simulink model "Demo_V2XStats_Intersection_1_cs"  (R2014b)
settings: Solver=FixedStepDiscrete  SolverMode=SingleTasking  StartTime=0.0  StopTime=10  FixedStep=1/20  RelTol=1e-3
PreLoadFcn:
  | mbxruntime.callbacks.PreLoadFcn(bdroot);
  | check_NUTS_defined
  | model_closed = 0;
  | assignin('base',['model_closed_' bdroot],false);
PostLoadFcn:
  | mbxruntime.callbacks.PostLoadFcn(bdroot);
InitFcn:
  | mbxruntime.callbacks.InitFcn(bdroot);
StartFcn:
  | mbxruntime.callbacks.StartFcn(bdroot);
StopFcn:
  | mbxruntime.callbacks.StopFcn(bdroot);;
  | 
  | PostProcessing
  | 
model workspace: external: MAT-File .\Demo_V2XStats_Intersection_1_cs_hws.mat (data not in the file)
undefined symbols (not defined in the file or in its folder): InitializeBus, mbxruntime, tabledata
undefined symbols (not defined in the file): Demo_V2XStats_Intersection_1_cs_022fa72960d02a99, Demo_V2XStats_Intersection_1_cs_0667b7440011464a, Demo_V2XStats_Intersection_1_cs_0a717f3b1f82dce8, Demo_V2XStats_Intersection_1_cs_1912d0ac773e0614, Demo_V2XStats_Intersection_1_cs_1b4820430dd12493, Demo_V2XStats_Intersection_1_cs_3bba87328ee67e0a, Demo_V2XStats_Intersection_1_cs_467d7b57b3557fc2, Demo_V2XStats_Intersection_1_cs_534bad308c560994, Demo_V2XStats_Intersection_1_cs_58d6839509a0e403, Demo_V2XStats_Intersection_1_cs_7e2090151d7b4087, Demo_V2XStats_Intersection_1_cs_9888c4f7e8bf41a4, Demo_V2XStats_Intersection_1_cs_a103b1f27004d7b9, Demo_V2XStats_Intersection_1_cs_dde6e9b2bb85eae6, Demo_V2XStats_Intersection_1_cs_fcdd4688b7d5d124
libraries: simulink x5, PreScanSimulinkLibrary x4, PreScanUsefulBlocks x1, simulink_extras x1
(part 1 of 3)
CloseFcn:
  | mbxruntime.callbacks.CloseFcn(bdroot);
  | evalin('base',['clear model_closed_' bdroot]);
  | model_closed = 1;
settings Model: Creator=PRESCAN  LastModifiedBy=stq0ee
settings DataIOCC: SignalLoggingSaveFormat=ModelDataLogs
settings OptimizationCC: InlineParams=on  ExpressionDepthLimit=2147483647  InitFltsAndDblsToZero=on
settings DebuggingCC: SaveWithParameterizedLinksMsg=none  UnderspecifiedInitializationDetection=Classic  MergeDetectMultiDrivingBlocksExec=none  SignalResolutionControl=TryResolveAllWithWarning  SolverPrmCheckMsg=none  MultiTaskDSMMsg=warning  MultiTaskCondExecSysMsg=none  FcnCallInpInsideContextMsg=UseLocalSettings  StateNameClashWarn=warning
settings ModelReferenceCC: UpdateModelReferenceTargets=IfOutOfDate
settings SFSimCC: SimParseCustomCode=off
settings SFSimCC: SimCustomHeaderCode=|
  | #include "prescan.h"
  | #include "prescan_platform.h"
  | #include "prescan_v2x_data.h"
settings RTWCC: IncludeERTFirstTime=on
settings GRTTargetCC: TargetFcnLib=ansi_tfl_tmw.mat  CombineOutputUpdateFcns=off  GRTInterface=on

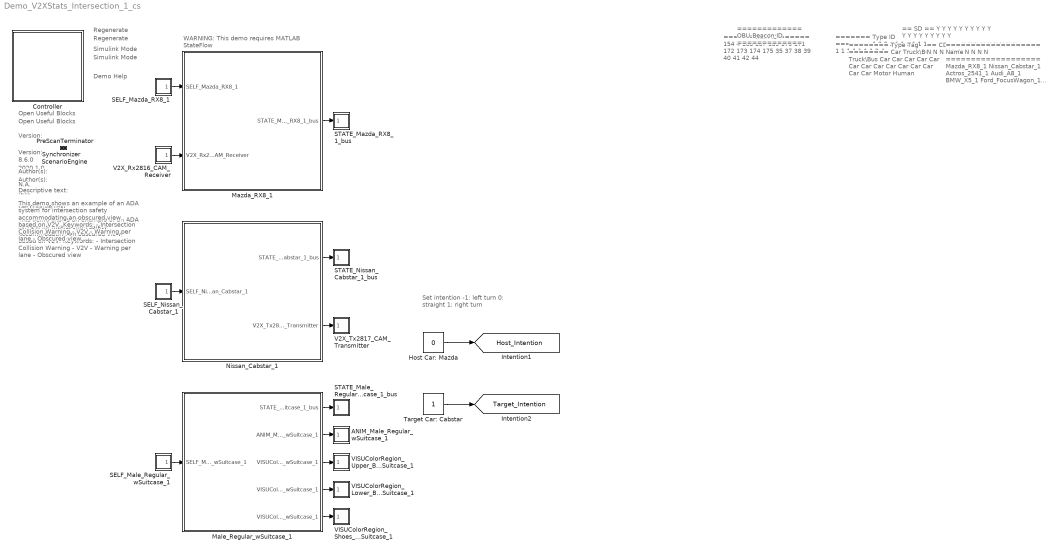
== system Demo_V2XStats_Intersection_1_cs ==
  note: Regenerate
  note: Simulink Mode
  note: Open Useful Blocks
  note: 2020.1.0
  note: Version:
  note: Author(s):
  note: N.A.
  note: Descriptive text:
  note: This demo shows an example of an
      | ADA system for intersection
      | safety accommodating an obscured
      | view, based on V2V.
      |
      |
      |
      | Keywords:
      |
      | - Intersection Collision Warning
      |
      | - V2V
      |
      | - Warning per lane
      |
      | - Obscured view
  note: 8.6.0
  note: Demo Help
  note: WARNING:
      | This demo requires MATLAB StateFlow
  note: Set intention
      | -1: left turn
      | 0: straight
      | 1: right turn
  note: This demo shows an example of an
      | ADA system for intersection
      | safety accommodating an obscured
      | view, based on V2V.
      |
      |
      |
      | Keywords:
      |
      | - Intersection Collision Warning
      |
      | - V2V
      |
      | - Warning per lane
      |
      | - Obscured view
  note: Descriptive text:
  note: N.A.
  note: Author(s):
  note: Version:
  note: Open Useful Blocks
  note: Simulink Mode
  note: Regenerate
  note: ======
      | Num ID
      | ======
      | 154
      | 4
      | 168
      | 167
      | 169
      | 170
      | 171
      | 172
      | 173
      | 174
      | 175
      | 35
      | 37
      | 38
      | 39
      | 40
      | 41
      | 42
      | 44
  note: =============
      | OBU-Beacon ID
      | =============
  note: =======
      | Type ID
      | =======
      | 1
      | 3
      | 3
      | 1
      | 1
      | 1
      | 1
      | 1
      | 1
      | 1
      | 1
      | 1
      | 1
      | 1
      | 1
      | 1
      | 1
      | 2
      | 4
  note: ========
      | Type Tag
      | ========
      | Car
      | Truck\Bus
      | Truck\Bus
      | Car
      | Car
      | Car
      | Car
      | Car
      | Car
      | Car
      | Car
      | Car
      | Car
      | Car
      | Car
      | Car
      | Car
      | Motor
      | Human
  note: ==
      | SD
      | ==
      | Y
      | Y
      | Y
      | Y
      | Y
      | Y
      | Y
      | Y
      | Y
      | Y
      | Y
      | Y
      | Y
      | Y
      | Y
      | Y
      | Y
      | Y
      | Y
  note: ==
      | CD
      | ==
      | N
      | N
      | N
      | N
      | N
      | N
      | N
      | N
      | N
      | N
      | N
      | N
      | N
      | N
      | N
      | N
      | N
      | N
      | N
  note: ===================
      | Name
      | ===================
      | Mazda_RX8_1
      | Nissan_Cabstar_1
      | Actros_2541_1
      | Audi_A8_1
      | BMW_X5_1
      | Ford_FocusWagon_1
      | Fiat_Bravo_1
      | Toyota_Previa_2
      | Citroen_C3_1
      | BMW_Z3_1
      | Ford_FocusWagon_2
      | Audi_A8_2
      | BMW_X5_2
      | Ford_FocusWagon_3
      | Mazda_RX8_2
      | Mazda_RX8_3
      | Ford_Fiesta_1
      | Honda_Pan_European_1
      | Male_Regular_wSuitcase_1
  ANIM_Male_Regular_wSuitcase_1 : Subsystem  Tag=actuator/AnimationOutport  Priority=0  LoadFcn=load('PreScanAnimActuatorData.mat')  mask(PreScan Sink Block: State Animation){}
      mask help: The Human Animation port allows the human to walk, run or bend
      settings: OpenFcn=open_system([gcb '/Actuator'],'mask')
      mask Help: eval('openHelp(239)')
      mask Display: image(imread('HumanAnimated.jpg'))
  Controller : Subsystem  Description=8A3CD2955739A82C886C20AE3E253D78460D53180EE2C1B14CC08DF75A70BE77  Priority=-1  LoadFcn=load PreScanControllerData  mask(PreScan Simulation Controller){prescanversion='2020.1.0', ModelReferencing=off, TimeStep=1/20, ControlMode=0, PreScanExecutionMode=on, ControllerCount=0, ControllerIndex=0, ControllerOptions=''}
      mask prompts: prescanversion "PreScan Version"; ModelReferencing "Use Model Referencing"; TimeStep "Upload Period [s]"; ControlMode "Control Mode"; PreScanExecutionMode "Execution Mode"; ControllerCount "Controller Count"; ControllerIndex "Controller Index"; ControllerOptions "Controller Options"
      mask help:
      | Please do not remove this block from the compilation sheet,
      | as it connects the model to the PreScan environment.
      mask init:
      | model = bdroot(gcb);
      | ExperimentFile = mbxruntime.findExperimentFile(model,true); %relative path
      | 
      | [d1, d2, d3, prescandata] = prescan_Settings();
      | ModelDepo = fullfile(prescandata,'ModelDepo'); 
      | 
      | RTmode = mbxruntime.getRTMode(model);
      | 
      | SimulationMode = get_param(bdroot,'SimulationMode');
      | if strcmp(SimulationMode, 'rapid-accelerator')
      |     SimulationMode = 'external';
      | end
      | TargetName = get_param(bdroot,'SystemTargetFile');
      settings: ModelCloseFcn=assignin('base',['model_closed_' bdroot],true);
      mask Help: eval('openHelp(812)')
      mask Display: image(imread('prescanlogo.ico'))
  Host Car: Mazda : Constant  Value=0
  Male_Regular_wSuitcase_1 : Subsystem  Tag=WorldObjectSubSystem  InitFcn=UniqueId = '2658';
      mask init:
      | modelPath = GenericModelHelper.getGenericModelFilePath('ModelDepo','Humans\MaleSuitcase\Male_wSuitcase.pgmb','86bcb677b51d2887e0050f1727544e76');imagePath = GenericModelHelper.getCompilationPicture(modelPath, 'MaleSuitcase.png');
      mask Display: image(imread(imagePath));color('white');text(0, 0, ' ID=44\n')
  Mazda_RX8_1 : Subsystem  Tag=WorldObjectSubSystem  InitFcn=UniqueId = '7';
      mask init:
      | modelPath = GenericModelHelper.getGenericModelFilePath('ModelDepo','Vehicles\Mazda_RX8\Mazda_RX8.pgmb','1e55a2e40efa576b7f4fb93bae35d605');imagePath = GenericModelHelper.getCompilationPicture(modelPath, 'Mazda_RX8_HighPoly.png');
      mask Display: image(imread(imagePath));color('white');text(0, 0, ' ID=154\n')
  Nissan_Cabstar_1 : Subsystem  Tag=WorldObjectSubSystem  InitFcn=UniqueId = '10';
      mask init:
      | modelPath = GenericModelHelper.getGenericModelFilePath('ModelDepo','Vehicles\Nissan_Cabstar\Nissan_Cabstar.pgmb','dd076fdae311093c5436e82e6c23dc23');imagePath = GenericModelHelper.getCompilationPicture(modelPath, 'Nissan_Cabstar_HighPoly.png');
      mask Display: image(imread(imagePath));color('white');text(0, 0, ' ID=4\n')
  PreScanTerminator : Subsystem  Tag=PreScanTerminator  Priority=999  LoadFcn=load PrescanTerminatorData  mask(PreScan Simulation Terminator){TimeStep=1/20}
      mask prompts: TimeStep "Upload Period [s]"
      mask help:
      | Please do not remove this block from the compilation sheet as it
      | connects the model to the PreScan environment.
      mask Help: eval('openHelp(812)')
      mask Display: image(imread('prescanlogo.ico'))
  SELF_Male_Regular_wSuitcase_1 : Subsystem  Tag=sensor/SelfPort  Priority=30  LoadFcn=load('PreScanSelfSensorData.mat')  mask(PreScan Source Block: SELF){}
      mask help:
      | The SELF port shows (state) information of the actor itself. The outputs are position in the experiment's axis system and the GPS coordinates, and the object's absolute velocity and compass heading.
      |
      | For more information, please click Help.
      settings: OpenFcn=open_system([gcb '/Sensor'],'mask')
      mask Help: eval('openHelp(462)')
      mask Display: image(imread('GPS.png'))
  SELF_Mazda_RX8_1 : Subsystem  Tag=sensor/SelfPort  Priority=30  LoadFcn=load('PreScanSelfSensorData.mat')  mask(PreScan Source Block: SELF){}
      mask help:
      | The SELF port shows (state) information of the actor itself. The outputs are position in the experiment's axis system and the GPS coordinates, and the object's absolute velocity and compass heading.
      |
      | For more information, please click Help.
      settings: OpenFcn=open_system([gcb '/Sensor'],'mask')
      mask Help: eval('openHelp(462)')
      mask Display: image(imread('GPS.png'))
  SELF_Nissan_Cabstar_1 : Subsystem  Tag=sensor/SelfPort  Priority=30  LoadFcn=load('PreScanSelfSensorData.mat')  mask(PreScan Source Block: SELF){}
      mask help:
      | The SELF port shows (state) information of the actor itself. The outputs are position in the experiment's axis system and the GPS coordinates, and the object's absolute velocity and compass heading.
      |
      | For more information, please click Help.
      settings: OpenFcn=open_system([gcb '/Sensor'],'mask')
      mask Help: eval('openHelp(462)')
      mask Display: image(imread('GPS.png'))
  STATE_Male_Regular_wSuitcase_1_bus : Subsystem  Tag=actuator/StatePort  Priority=0  LoadFcn=load('PreScanStateActuatorData.mat')  mask(PreScan Sink Block: State){}
      mask help:
      | The Actor State contains a vector signal of size (9x1), containing the following signals:
      |
      | -  Position    	(x,y,z)             	[m]
      | -  Velocity    	(vx,vy,vz)         	[m/s]
      | -  Angles       	(Roll, Pitch, Yaw)	[rad]
      |
      | The Actor state is defined in the global axis system.
      | The state is superponed on the Initial position defined in the GUI.
      |
      | For more information, please click Help.
      settings: OpenFcn=open_system([gcb '/Actuator'],'mask')
      mask Help: eval('openHelp(222)')
      mask Display: image(imread('State.png'))
  STATE_Mazda_RX8_1_bus : Subsystem  Tag=actuator/StatePort  Priority=0  LoadFcn=load('PreScanStateActuatorData.mat')  mask(PreScan Sink Block: State){}
      mask help:
      | The Actor State contains a vector signal of size (9x1), containing the following signals:
      |
      | -  Position    	(x,y,z)             	[m]
      | -  Velocity    	(vx,vy,vz)         	[m/s]
      | -  Angles       	(Roll, Pitch, Yaw)	[rad]
      |
      | The Actor state is defined in the global axis system.
      | The state is superponed on the Initial position defined in the GUI.
      |
      | For more information, please click Help.
      settings: OpenFcn=open_system([gcb '/Actuator'],'mask')
      mask Help: eval('openHelp(222)')
      mask Display: image(imread('State.png'))
  STATE_Nissan_Cabstar_1_bus : Subsystem  Tag=actuator/StatePort  Priority=0  LoadFcn=load('PreScanStateActuatorData.mat')  mask(PreScan Sink Block: State){}
      mask help:
      | The Actor State contains a vector signal of size (9x1), containing the following signals:
      |
      | -  Position    	(x,y,z)             	[m]
      | -  Velocity    	(vx,vy,vz)         	[m/s]
      | -  Angles       	(Roll, Pitch, Yaw)	[rad]
      |
      | The Actor state is defined in the global axis system.
      | The state is superponed on the Initial position defined in the GUI.
      |
      | For more information, please click Help.
      settings: OpenFcn=open_system([gcb '/Actuator'],'mask')
      mask Help: eval('openHelp(222)')
      mask Display: image(imread('State.png'))
  ScenarioEngine : Subsystem  Tag=PreScanOpenScenarioBlock  Priority=10  LoadFcn=load PrescanSynchronizeData  mask(PreScan Simulation Core Block){TimeStep=1/20}
      mask prompts: TimeStep "Timestep [s]"
      mask help:
      | Please do not remove this block from the PreScan compilation sheet,
      | as it contains essential configuration parameters for a PreScan simulation.
      settings: DeleteFcn=PreScanBlockDeleteFcn;
      mask Display: image(imread('prescanlogo.ico'))
  Synchronizer : Subsystem  Tag=PreScanSynchronizer  Priority=20  LoadFcn=load PrescanSynchronizeData  mask(PreScan Simulation Core Block){TimeStep=1/20}
      mask prompts: TimeStep "Timestep [s]"
      mask help:
      | Please do not remove this block from the PreScan compilation sheet,
      | as it contains essential configuration parameters for a PreScan simulation.
      settings: DeleteFcn=PreScanBlockDeleteFcn;
      mask Display: image(imread('prescanlogo.ico'))
  Target Car: Cabstar : Constant
  V2X_Rx2816_CAM_Receiver : Subsystem  Tag=sensor/plugin/sfun_V2X_CAM_Receiver  Priority=30  mask(V2X CAM Receiver Block){}
      mask help: V2X Block receiving a CAM message
      settings: OpenFcn=open_system([gcb '/Sensor'],'mask')
      mask Help: eval('openHelp()')
      mask Display: image(imread('V2XR_grayscale.png'))
  V2X_Tx2817_CAM_Transmitter : Subsystem  Tag=actuator/plugin/sfun_V2X_CAM_Transmitter  Priority=0  mask(V2X CAM Transmitter Block){}
      mask help: V2X Block transmitting a CAM message
      settings: OpenFcn=open_system([gcb '/Actuator'],'mask')
      mask Help: eval('openHelp()')
      mask Display: image(imread('V2XT_grayscale.png'))
  VISUColorRegion_Lower_Body_Male_Regular_wSuitcase_1 : Subsystem  Tag=actuator/ColorRegion  Priority=0  LoadFcn=load('PrescanColorData')  mask(PreScan Sink Block: VisuTextureColor){}
      mask help:
      | The VisuTextureColor block provides a way to adapt the color of a vehicle.
      |
      | For more information, please click Help.
      settings: OpenFcn=open_system([gcb '/Actuator'],'mask')
      mask Help: eval('openHelp(230)')
      mask Display: image(imread('TextureColor.png'))
  VISUColorRegion_Shoes_Male_Regular_wSuitcase_1 : Subsystem  Tag=actuator/ColorRegion  Priority=0  LoadFcn=load('PrescanColorData')  mask(PreScan Sink Block: VisuTextureColor){}
      mask help:
      | The VisuTextureColor block provides a way to adapt the color of a vehicle.
      |
      | For more information, please click Help.
      settings: OpenFcn=open_system([gcb '/Actuator'],'mask')
      mask Help: eval('openHelp(230)')
      mask Display: image(imread('TextureColor.png'))
  VISUColorRegion_Upper_Body_Male_Regular_wSuitcase_1 : Subsystem  Tag=actuator/ColorRegion  Priority=0  LoadFcn=load('PrescanColorData')  mask(PreScan Sink Block: VisuTextureColor){}
      mask help:
      | The VisuTextureColor block provides a way to adapt the color of a vehicle.
      |
      | For more information, please click Help.
      settings: OpenFcn=open_system([gcb '/Actuator'],'mask')
      mask Help: eval('openHelp(230)')
      mask Display: image(imread('TextureColor.png'))
  tag scope: Host_Intention=global, Target_Intention=global
  wires:
  Host Car: Mazda/1 -> [Host_Intention]
  Target Car: Cabstar/1 -> [Target_Intention]
  SELF_Nissan_Cabstar_1/1(SELF_Nissan_Cabstar_1) -> Nissan_Cabstar_1/1(SELF_Nissan_Cabstar_1)
  Nissan_Cabstar_1/2(V2X_Tx2817_CAM_Transmitter) -> V2X_Tx2817_CAM_Transmitter/1(V2X_Tx2817_CAM_Transmitter)
  Nissan_Cabstar_1/1(STATE_Nissan_Cabstar_1_bus) -> STATE_Nissan_Cabstar_1_bus/1(STATE_Nissan_Cabstar_1_bus)
  V2X_Rx2816_CAM_Receiver/1(V2X_Rx2816_CAM_Receiver) -> Mazda_RX8_1/2(V2X_Rx2816_CAM_Receiver)
  SELF_Mazda_RX8_1/1(SELF_Mazda_RX8_1) -> Mazda_RX8_1/1(SELF_Mazda_RX8_1)
  Mazda_RX8_1/1(STATE_Mazda_RX8_1_bus) -> STATE_Mazda_RX8_1_bus/1(STATE_Mazda_RX8_1_bus)
  SELF_Male_Regular_wSuitcase_1/1(SELF_Male_Regular_wSuitcase_1) -> Male_Regular_wSuitcase_1/1(SELF_Male_Regular_wSuitcase_1)
  Male_Regular_wSuitcase_1/2(ANIM_Male_Regular_wSuitcase_1) -> ANIM_Male_Regular_wSuitcase_1/1(ANIM_Male_Regular_wSuitcase_1)
  Male_Regular_wSuitcase_1/1(STATE_Male_Regular_wSuitcase_1_bus) -> STATE_Male_Regular_wSuitcase_1_bus/1(STATE_Male_Regular_wSuitcase_1_bus)
  Male_Regular_wSuitcase_1/3(VISUColorRegion_Upper_Body_Male_Regular_wSuitcase_1) -> VISUColorRegion_Upper_Body_Male_Regular_wSuitcase_1/1(VISUColorRegion_Upper_Body_Male_Regular_wSuitcase_1)
  Male_Regular_wSuitcase_1/4(VISUColorRegion_Lower_Body_Male_Regular_wSuitcase_1) -> VISUColorRegion_Lower_Body_Male_Regular_wSuitcase_1/1(VISUColorRegion_Lower_Body_Male_Regular_wSuitcase_1)
  Male_Regular_wSuitcase_1/5(VISUColorRegion_Shoes_Male_Regular_wSuitcase_1) -> VISUColorRegion_Shoes_Male_Regular_wSuitcase_1/1(VISUColorRegion_Shoes_Male_Regular_wSuitcase_1)

== system Demo_V2XStats_Intersection_1_cs/ANIM_Male_Regular_wSuitcase_1 ==
  ANIM_Male_Regular_wSuitcase_1 : Inport  Tag=inport/AnimationOutport  OutDataTypeStr=Bus: PRESCAN_ANIMACTUATORDATA  PortDimensions=1  SampleTime=1/20  BusOutputAsStruct=on
  Actuator : S-Function  FunctionName=sfun_AnimActuator  Parameters=UniqueID, TimeStep  EnableBusSupport=off  mask(PreScan Sink Block: State Animation){UniqueID=2658, TimeStep=1/20}
      mask prompts: UniqueID "Auto-Assigned: Unique ID"; TimeStep "Auto-Assigned: Upload Period [s]"
      mask help: The Human Animation port allows the human to walk, run or bend
      mask Help: eval('openHelp(239)')
      mask Display: image(imread('HumanAnimated.jpg'))
  wires:
  ANIM_Male_Regular_wSuitcase_1/1 -> Actuator/1

== system Demo_V2XStats_Intersection_1_cs/Controller ==
  Terminator : Terminator
  sfun_Controller : S-Function  FunctionName=sfun_Controller  Parameters=SParameter1, SParameter2, SParameter3, SParameter4, SParameter5, SParameter6, SParameter7, SParameter8, SParameter9, SParameter10, SampleTime  EnableBusSupport=off  mask(Legacy Function){SFunctionSpec=void prescan_outputFcn(void** work1, PRESCAN_CONTROLLERDATA y1[1]), SParameter1=uint8([ExperimentFile 0]), SParameter2=uint8([ModelDepo 0]), SParameter3=uint8([ControllerOptions 0]), SParameter4=RTmode, SParameter5=PreScanExecutionMode, SParameter6=ControlMode, SParameter7=ControllerCount, SParameter8=ControllerIndex, SParameter9=uint8([SimulationMode 0]), SParameter10=uint8([TargetName 0]), SampleTime=TimeStep, ShowSpec=on}
      mask prompts: SParameter1 "P1:"; SParameter2 "P2:"; SParameter3 "P3:"; SParameter4 "P4:"; SParameter5 "P5:"; SParameter6 "P6:"; SParameter7 "P7:"; SParameter8 "P8:"; SParameter9 "P9:"; SParameter10 "P10:"; SampleTime "Sample time (-1 for inherited):"; ShowSpec "Display function specification"
      mask help:
      | This block allows you to call the legacy functions specified by the following Legacy Code Tool definition:
      | def.SFunctionName = 'sfun_Controller';
      | def.OutputFcnSpec = 'void prescan_outputFcn(void** work1, PRESCAN_CONTROLLERDATA y1[1])';
      | def.StartFcnSpec = 'void prescan_startFcn(void ** work1, uint8 p1[], uint8 p2[], uint8 p3[], double p4, double p5, double p6, double p7, double p8, uint8 p9[], uint8 p10[])';
      | def.TerminateFcnSpec = 'void prescan_terminateFcn(void** work1)';
      | def.HeaderFiles = {'prescan_controller_data.h', 'prescan_SFunLibrary.h', 'prescan_CreateLogHandler.h', 'prescan_CreateErrorHandler.h', 'prescan_modify.h', 'ModuleDLL.h'};
      | def.SourceFiles = {'prescan_MexLogHandler.c', 'prescan_SimStructErrorHandler.c', 'prescan_LogHandler.c', 'prescan_ErrorHandler.c', 'prescan_Modify.c'};
      | def.HostLibFiles = {'sensorinterfaced.lib'};
      | def.TargetLibFiles = {'sensorinterfaced.so'};
      | def.IncPaths = {'.', 'C:\projects\prescan\rt_vislibrary\vis\..\pimp\include\sensors\InterfaceRTW'};
      | def.SrcPaths = {'C:\projects\prescan\rt_vislibrary\vis\..\pimp\include\sensors\InterfaceRTW', 'C:\projects\prescan\rt_vislibrary\vis\..\pimp\include\sensors\InterfaceRTW\ccurrt'};
      | def.LibPaths = {'C:\\projects\\prescan\\vislibrary_build\lib'};
      | def.SampleTime = 'parameterized';
      mask Help: <p>This block was generated automatically by the Legacy Code Tool. For detailed help on this tool, call<a href="matlab:legacy_code('help')"> legacy_code('help')</a>.</p>
      mask Callback ShowSpec:
      | if strcmp(get_param(gcbh, 'ShowSpec'), 'on')
      |   set_param(gcbh, 'MaskDisplay', sprintf('fprintf(''%s'');', get_param(gcbh, 'SFunctionSpec')));
      | else
      |   set_param(gcbh, 'MaskDisplay', sprintf('fprintf(''%s'');', get_param(gcbh, 'FunctionName')));
      | end
      mask Display: fprintf('void prescan_outputFcn(void** work1, PRESCAN_CONTROLLERDATA y1[1])');
  wires:
  sfun_Controller/1 -> Terminator/1

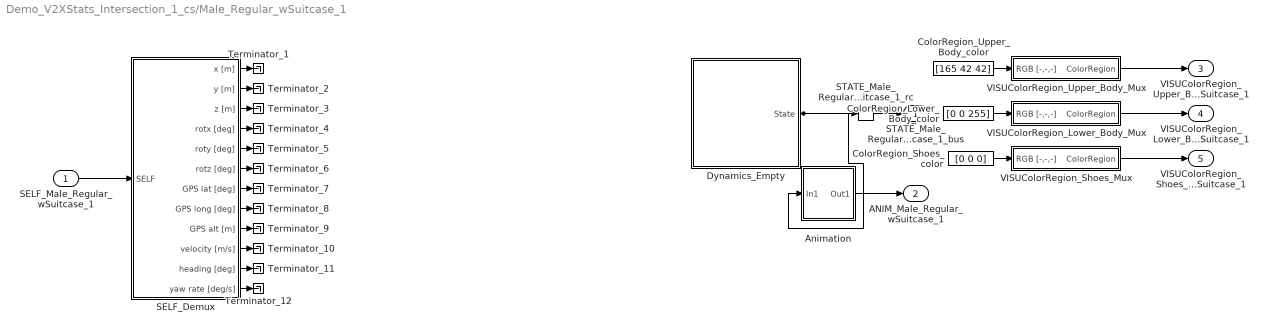
== system Demo_V2XStats_Intersection_1_cs/Male_Regular_wSuitcase_1 ==
  SELF_Male_Regular_wSuitcase_1 : Inport  Tag=inport/SelfPort  OutDataTypeStr=Bus: PRESCAN_SELFSENSORDATA  PortDimensions=1  SampleTime=1/20  BusOutputAsStruct=on
  Animation : Subsystem  Tag=WalkingHumanAnimation  mask(Prescan Conversion Block: Walking Human Animation){TimeStep=1/20}
      mask prompts: TimeStep "Auto-Assigned: Upload Period [s]"
      mask help: The Walking Human Animation block converts the State signal of a human into signals to properly control the animation.
      mask Help: eval('openHelp(239)');
      mask Display: image(imread('HumanAnimated.jpg'))
  ColorRegion_Lower_Body_color : Constant  Tag=VisuLightConst  Value=[0 0 255]
  ColorRegion_Shoes_color : Constant  Tag=VisuLightConst  Value=[0 0 0]
  ColorRegion_Upper_Body_color : Constant  Tag=VisuLightConst  Value=[165 42 42]
  Dynamics_Empty : Subsystem  Tag=Dynamics_Empty
      mask Help: eval('openHelp(202)')
      mask Display: port_label('output', 1, 'State');text(0,0,' Empty\n')
  SELF_Demux : Subsystem  Tag=demux/SelfPort  mask(PreScan Demux Block:){}
      mask help:
      | The SELF port shows (state) information of the actor itself. The outputs are position in the experiment's axis system and the GPS coordinates, and the object's absolute velocity and compass heading.
      |
      | For more information, please click Help.
      settings: DeleteFcn=PreScanBlockDeleteFcn;
      mask Help: eval('openHelp(462)')
      mask Display:
      | port_label('output',1,'x [m]')
      | port_label('output',2,'y [m]')
      | port_label('output',3,'z [m]','texmode','on')
      | port_label('output',4,'Rotx [deg]','texmode','on')
      | port_label('output',5,'Roty [deg]','texmode','on')
      | port_label('output',6,'Rotz [deg]','texmode','on')
      | port_label('output',7,'GPS lat [deg]','texmode','on')
      | port_label('output',8,'GPS long [deg]','texmode','on')
      | port_label('output',9,'GPS alt [m]','texmode','on')
      | port_label('output',10,'Velocity [m/s]')
      | port_label('output',11,'Heading [deg]')
      | port_label('output',12,'Yaw rate [deg/s]')
  STATE_Male_Regular_wSuitcase_1_rc : RateTransition  Tag=mux_rc/StatePort  OutPortSampleTimeOpt=Inherit
  Terminator_{1..12} (12 alike) : Terminator
  VISUColorRegion_Lower_Body_Mux : Subsystem  Tag=mux/MuxColorRegion  LoadFcn=load PrescanColorData  mask(PreScan User Interface: VisuTextureColor){}
      mask help:
      | The VisuTextureColor block provides a way to adapt the color of a vehicle.
      |
      | For more information, please click Help.
      settings: DeleteFcn=PreScanBlockDeleteFcn;
      mask Help: eval('openHelp(230)')
  VISUColorRegion_Shoes_Mux : Subsystem  Tag=mux/MuxColorRegion  LoadFcn=load PrescanColorData  mask(PreScan User Interface: VisuTextureColor){}
      mask help:
      | The VisuTextureColor block provides a way to adapt the color of a vehicle.
      |
      | For more information, please click Help.
      settings: DeleteFcn=PreScanBlockDeleteFcn;
      mask Help: eval('openHelp(230)')
  VISUColorRegion_Upper_Body_Mux : Subsystem  Tag=mux/MuxColorRegion  LoadFcn=load PrescanColorData  mask(PreScan User Interface: VisuTextureColor){}
      mask help:
      | The VisuTextureColor block provides a way to adapt the color of a vehicle.
      |
      | For more information, please click Help.
      settings: DeleteFcn=PreScanBlockDeleteFcn;
      mask Help: eval('openHelp(230)')
  STATE_Male_Regular_wSuitcase_1_bus : Outport  Tag=outport/StatePort  OutDataTypeStr=Bus: PRESCAN_STATEACTUATORDATA  PortDimensions=1  SampleTime=1/20
  ANIM_Male_Regular_wSuitcase_1 : Outport  Tag=outport/AnimationOutport  Port=2  OutDataTypeStr=Bus: PRESCAN_ANIMACTUATORDATA  PortDimensions=1  SampleTime=1/20
  VISUColorRegion_Upper_Body_Male_Regular_wSuitcase_1 : Outport  Tag=outport/ColorRegion  Port=3  OutDataTypeStr=Bus: PRESCAN_COLOR_DATA  PortDimensions=1  SampleTime=1/20
  VISUColorRegion_Lower_Body_Male_Regular_wSuitcase_1 : Outport  Tag=outport/ColorRegion  Port=4  OutDataTypeStr=Bus: PRESCAN_COLOR_DATA  PortDimensions=1  SampleTime=1/20
  VISUColorRegion_Shoes_Male_Regular_wSuitcase_1 : Outport  Tag=outport/ColorRegion  Port=5  OutDataTypeStr=Bus: PRESCAN_COLOR_DATA  PortDimensions=1  SampleTime=1/20
  wires:
  STATE_Male_Regular_wSuitcase_1_rc/1 -> STATE_Male_Regular_wSuitcase_1_bus/1
  Dynamics_Empty/1(State) -> STATE_Male_Regular_wSuitcase_1_rc/1, Animation/1(In1)
  Animation/1(Out1) -> ANIM_Male_Regular_wSuitcase_1/1
  SELF_Male_Regular_wSuitcase_1/1 -> SELF_Demux/1(SELF)
  VISUColorRegion_Upper_Body_Mux/1(ColorRegion) -> VISUColorRegion_Upper_Body_Male_Regular_wSuitcase_1/1
  ColorRegion_Upper_Body_color/1 -> VISUColorRegion_Upper_Body_Mux/1(RGB [-,-,-])
  VISUColorRegion_Lower_Body_Mux/1(ColorRegion) -> VISUColorRegion_Lower_Body_Male_Regular_wSuitcase_1/1
  ColorRegion_Lower_Body_color/1 -> VISUColorRegion_Lower_Body_Mux/1(RGB [-,-,-])
  VISUColorRegion_Shoes_Mux/1(ColorRegion) -> VISUColorRegion_Shoes_Male_Regular_wSuitcase_1/1
  ColorRegion_Shoes_color/1 -> VISUColorRegion_Shoes_Mux/1(RGB [-,-,-])
  SELF_Demux/1(x [m]) -> Terminator_1/1
  SELF_Demux/2(y [m]) -> Terminator_2/1
  SELF_Demux/3(z [m]) -> Terminator_3/1
  SELF_Demux/4(rotx [deg]) -> Terminator_4/1
  SELF_Demux/5(roty [deg]) -> Terminator_5/1
  SELF_Demux/6(rotz [deg]) -> Terminator_6/1
  SELF_Demux/7(GPS lat [deg]) -> Terminator_7/1
  SELF_Demux/8(GPS long [deg]) -> Terminator_8/1
  SELF_Demux/9(GPS alt [m]) -> Terminator_9/1
  SELF_Demux/10(velocity [m/s]) -> Terminator_10/1
  SELF_Demux/11(heading [deg]) -> Terminator_11/1
  SELF_Demux/12(yaw rate [deg/s]) -> Terminator_12/1

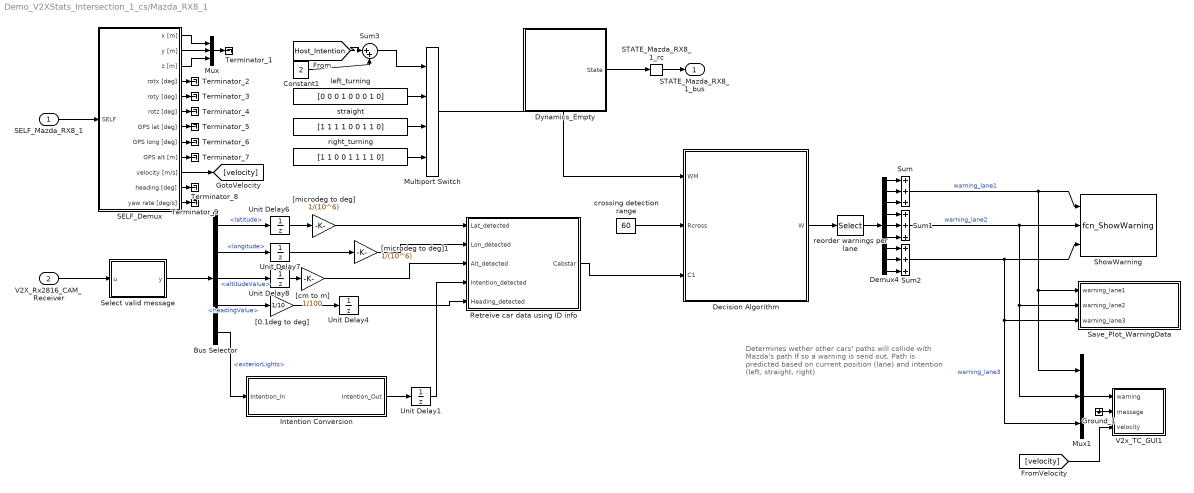
== system Demo_V2XStats_Intersection_1_cs/Mazda_RX8_1 ==
  note: Determines wether other cars' paths
      | will collide with Mazda's path
      | If so a warning is send out.
      |
      | Path is predicted based on current position (lane)
      | and intention (left, straight, right)
  SELF_Mazda_RX8_1 : Inport  Tag=inport/SelfPort  OutDataTypeStr=Bus: PRESCAN_SELFSENSORDATA  PortDimensions=1  SampleTime=1/20  BusOutputAsStruct=on
  V2X_Rx2816_CAM_Receiver : Inport  Tag=inport/plugin/sfun_V2X_CAM_Receiver  Port=2  BusOutputAsStruct=on
  Bus Selector : BusSelector  OutputSignals=DATA.cam.camParameters.basicContainer.referencePosition.latitude,DATA.cam.camParameters.basicContainer.referencePosition.longitude,DATA.cam.camParameters.basicContainer.referencePosition.altitude.altitudeValue,DATA.cam.camParameters.highFrequencyContainer.basicVehicleContainerHighFrequency.heading.headingValue,DATA.cam.camParameters.lowFrequencyContainer.basicVehicleContainerLowFrequency.exteriorLights
  Constant1 : Constant  Value=2
  Decision Algorithm : Stateflow chart  TreatAsAtomicUnit=on
  Demux4 : Demux  Outputs=9
  Dynamics_Empty : Subsystem  Tag=Dynamics_Empty
      mask Help: eval('openHelp(202)')
      mask Display: port_label('output', 1, 'State');text(0,0,' Empty\n')
  Ground_1 : Ground
  Intention Conversion : MATLAB Function  TreatAsAtomicUnit=on
  Multiport Switch : MultiPortSwitch
  Mux : Mux  Inputs=3
  Mux1 : Mux  Inputs=3
  Retreive car data using ID info : Subsystem
  SELF_Demux : Subsystem  Tag=demux/SelfPort  mask(PreScan Demux Block:){}
      mask help:
      | The SELF port shows (state) information of the actor itself. The outputs are position in the experiment's axis system and the GPS coordinates, and the object's absolute velocity and compass heading.
      |
      | For more information, please click Help.
      settings: DeleteFcn=PreScanBlockDeleteFcn;
      mask Help: eval('openHelp(462)')
      mask Display:
      | port_label('output',1,'x [m]')
      | port_label('output',2,'y [m]')
      | port_label('output',3,'z [m]','texmode','on')
      | port_label('output',4,'Rotx [deg]','texmode','on')
      | port_label('output',5,'Roty [deg]','texmode','on')
      | port_label('output',6,'Rotz [deg]','texmode','on')
      | port_label('output',7,'GPS lat [deg]','texmode','on')
      | port_label('output',8,'GPS long [deg]','texmode','on')
      | port_label('output',9,'GPS alt [m]','texmode','on')
      | port_label('output',10,'Velocity [m/s]')
      | port_label('output',11,'Heading [deg]')
      | port_label('output',12,'Yaw rate [deg/s]')
  STATE_Mazda_RX8_1_rc : RateTransition  Tag=mux_rc/StatePort  OutPortSampleTimeOpt=Inherit
  Save_Plot_WarningData : Subsystem
  Select valid message : MATLAB Function  TreatAsAtomicUnit=on
  ShowWarning : M-S-Function  FunctionName=fcn_ShowWarning  Parameters=ImageFile FigHandle WarningColor 1  mask{ImageFile='Mazda_RX8Top.png', FigHandle=10, WarningColor='y'}
      mask prompts: ImageFile "Image file"; FigHandle "Figure handle"
  Sum : Sum  Inputs=+++
  Sum1 : Sum  Inputs=+++
  Sum2 : Sum  Inputs=+++
  Sum3 : Sum  Inputs=|++
  Terminator_{1..9} (9 alike) : Terminator
  Unit Delay{1,4,6..8} (5 alike) : UnitDelay  SampleTime=-1
  V2x_TC_GUI1 : Subsystem
  "[0.1deg to deg]" : Gain  Gain=1/10  OutDataTypeStr=double
  "[cm to m]" : Gain  Gain=1/100  OutDataTypeStr=double
  "[microdeg to deg]" : Gain  Gain=1/(10^6)  OutDataTypeStr=double
  "[microdeg to deg]1" : Gain  Gain=1/(10^6)  OutDataTypeStr=double
  crossing detection range : Constant  Value=60
  left_turning : Constant  Value=[0 0 0 1 0 0 0 1 0]
  reorder warnings per lane : Selector  InputPortWidth=9  Indices=[1 4 7 2 5 8 3 6 9]
  right_turning : Constant  Value=[1 1 0 0 1 1 1 1 0]
  straight : Constant  Value=[1 1 1 1 0 0 1 1 0]
  STATE_Mazda_RX8_1_bus : Outport  Tag=outport/StatePort  OutDataTypeStr=Bus: PRESCAN_STATEACTUATORDATA  PortDimensions=1  SampleTime=1/20
  wires:
  Bus Selector/1 -> Unit Delay6/1  "<latitude>"
  Unit Delay6/1 -> "[microdeg to deg]"/1
  "[microdeg to deg]"/1 -> Retreive car data using ID info/1(Lat_detected)
  Retreive car data using ID info/1(Cabstar) -> Decision Algorithm/3(C1)
  Decision Algorithm/1(W) -> reorder warnings per lane/1
  reorder warnings per lane/1 -> Demux4/1
  Demux4/1 -> Sum/1
  Sum/1 -> Mux1/1, Save_Plot_WarningData/1(warning_lane1), ShowWarning/1  "warning_lane1"
  Mux1/1 -> V2x_TC_GUI1/1(warning)
  [velocity] -> V2x_TC_GUI1/3(velocity)
  Sum1/1 -> Mux1/2, Save_Plot_WarningData/2(warning_lane2), ShowWarning/2  "warning_lane2"
  Sum2/1 -> Mux1/3, Save_Plot_WarningData/3(warning_lane3), ShowWarning/3  "warning_lane3"
  Demux4/2 -> Sum/2
  Demux4/3 -> Sum/3
  Demux4/4 -> Sum1/1
  Demux4/5 -> Sum1/2
  Demux4/6 -> Sum1/3
  Demux4/7 -> Sum2/1
  Demux4/8 -> Sum2/2
  Demux4/9 -> Sum2/3
  Multiport Switch/1 -> Decision Algorithm/1(WM)
  Sum3/1 -> Multiport Switch/1
  [Host_Intention] -> Sum3/1
  Constant1/1 -> Sum3/2
  left_turning/1 -> Multiport Switch/2
  straight/1 -> Multiport Switch/3
  right_turning/1 -> Multiport Switch/4
  crossing detection range/1 -> Decision Algorithm/2(Rcross)
  "[microdeg to deg]1"/1 -> Retreive car data using ID info/2(Lon_detected)
  Unit Delay7/1 -> "[microdeg to deg]1"/1
  "[cm to m]"/1 -> Retreive car data using ID info/3(Alt_detected)
  Unit Delay8/1 -> "[cm to m]"/1
  Unit Delay1/1 -> Retreive car data using ID info/4(Intention_detected)
  Intention Conversion/1(Intention_Out) -> Unit Delay1/1
  Unit Delay4/1 -> Retreive car data using ID info/5(Heading_detected)
  "[0.1deg to deg]"/1 -> Unit Delay4/1
  Bus Selector/2 -> Unit Delay7/1  "<longitude>"
  Bus Selector/3 -> Unit Delay8/1  "<altitudeValue>"
  Bus Selector/4 -> "[0.1deg to deg]"/1  "<headingValue>"
  Bus Selector/5 -> Intention Conversion/1(Intention_In)  "<exteriorLights>"
  Select valid message/1(y) -> Bus Selector/1
  V2X_Rx2816_CAM_Receiver/1 -> Select valid message/1(u)
  SELF_Demux/10(velocity [m/s]) -> [velocity]
  SELF_Demux/1(x [m]) -> Mux/1
  SELF_Demux/2(y [m]) -> Mux/2
  SELF_Demux/3(z [m]) -> Mux/3
  STATE_Mazda_RX8_1_rc/1 -> STATE_Mazda_RX8_1_bus/1
  Dynamics_Empty/1(State) -> STATE_Mazda_RX8_1_rc/1
  SELF_Mazda_RX8_1/1 -> SELF_Demux/1(SELF)
  Mux/1 -> Terminator_1/1
  SELF_Demux/4(rotx [deg]) -> Terminator_2/1
  SELF_Demux/5(roty [deg]) -> Terminator_3/1
  SELF_Demux/6(rotz [deg]) -> Terminator_4/1
  SELF_Demux/7(GPS lat [deg]) -> Terminator_5/1
  SELF_Demux/8(GPS long [deg]) -> Terminator_6/1
  SELF_Demux/9(GPS alt [m]) -> Terminator_7/1
  SELF_Demux/11(heading [deg]) -> Terminator_8/1
  SELF_Demux/12(yaw rate [deg/s]) -> Terminator_9/1
  Ground_1/1 -> V2x_TC_GUI1/2(message)

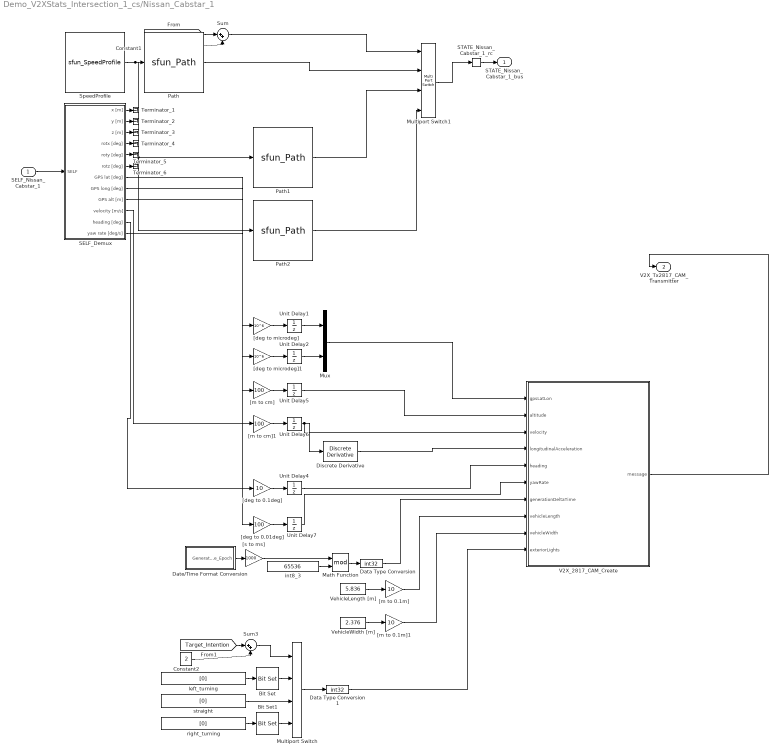
== system Demo_V2XStats_Intersection_1_cs/Nissan_Cabstar_1 ==
  SELF_Nissan_Cabstar_1 : Inport  Tag=inport/SelfPort  OutDataTypeStr=Bus: PRESCAN_SELFSENSORDATA  PortDimensions=1  SampleTime=1/20  BusOutputAsStruct=on
  Bit Set : simulink/Logic and Bit Operations/Bit Set  iBit=2
  Bit Set1 : simulink/Logic and Bit Operations/Bit Set  iBit=3
  Constant1 : Constant  Value=2
  Constant2 : Constant  Value=2
  Data Type Conversion : DataTypeConversion  OutDataTypeStr=int32
  Data Type Conversion1 : DataTypeConversion  OutDataTypeStr=int32
  Date/Time Format Conversion : MATLAB Function  TreatAsAtomicUnit=on
  Discrete Derivative : simulink/Discrete/Discrete Derivative  gainval=1.0  ICPrevScaledInput=0.0  InputProcessing=Inherited  OutMin=[]  OutMax=[]  OutDataTypeStr=int32  OutputDataTypeScalingMode=int32  OutDataType=fixdt(1, 16)  OutScaling=2^-10  DoSatur=off
  Math Function : Math  Operator=mod  SaturateOnIntegerOverflow=on
  Multiport Switch : MultiPortSwitch
  Multiport Switch1 : MultiPortSwitch
  Mux : Mux  Inputs=2
  Path : S-Function  Tag=Path  LoadFcn=load('PrescanMotionData.mat')  FunctionName=sfun_Path  Parameters=uniqueID, pathUniqueID, timestep  EnableBusSupport=off  mask(Path){uniqueID=10, pathUniqueID=Demo_V2XStats_Intersection_1_cs_a103b1f27004d7b9, timestep=1/20}
      mask prompts: uniqueID "Object Unique ID"; pathUniqueID "Path Unique ID"; timestep "MATLAB timestep:"
      mask help:
      | The path block outputs the position along a given trajectory.
      |
      | For more information, please click Help.
      mask Help: eval('openHelp(312)')
      mask Display: image(imread('Path.png'))
  Path1 : S-Function  Tag=Path  LoadFcn=load('PrescanMotionData.mat')  FunctionName=sfun_Path  Parameters=uniqueID, pathUniqueID, timestep  EnableBusSupport=off  mask(Path){uniqueID=10, pathUniqueID=59, timestep=1/20}
      mask prompts: uniqueID "Object Unique ID"; pathUniqueID "Path Unique ID"; timestep "MATLAB timestep:"
      mask help:
      | The path block outputs the position along a given trajectory.
      |
      | For more information, please click Help.
      mask Help: eval('openHelp(312)')
      mask Display: image(imread('Path.png'))
  Path2 : S-Function  Tag=Path  LoadFcn=load('PrescanMotionData.mat')  FunctionName=sfun_Path  Parameters=uniqueID, pathUniqueID, timestep  EnableBusSupport=off  mask(Path){uniqueID=10, pathUniqueID=60, timestep=1/20}
      mask prompts: uniqueID "Object Unique ID"; pathUniqueID "Path Unique ID"; timestep "MATLAB timestep:"
      mask help:
      | The path block outputs the position along a given trajectory.
      |
      | For more information, please click Help.
      mask Help: eval('openHelp(312)')
      mask Display: image(imread('Path.png'))
  SELF_Demux : Subsystem  Tag=demux/SelfPort  mask(PreScan Demux Block:){}
      mask help:
      | The SELF port shows (state) information of the actor itself. The outputs are position in the experiment's axis system and the GPS coordinates, and the object's absolute velocity and compass heading.
      |
      | For more information, please click Help.
      settings: DeleteFcn=PreScanBlockDeleteFcn;
      mask Help: eval('openHelp(462)')
      mask Display:
      | port_label('output',1,'x [m]')
      | port_label('output',2,'y [m]')
      | port_label('output',3,'z [m]','texmode','on')
      | port_label('output',4,'Rotx [deg]','texmode','on')
      | port_label('output',5,'Roty [deg]','texmode','on')
      | port_label('output',6,'Rotz [deg]','texmode','on')
      | port_label('output',7,'GPS lat [deg]','texmode','on')
      | port_label('output',8,'GPS long [deg]','texmode','on')
      | port_label('output',9,'GPS alt [m]','texmode','on')
      | port_label('output',10,'Velocity [m/s]')
      | port_label('output',11,'Heading [deg]')
      | port_label('output',12,'Yaw rate [deg/s]')
  STATE_Nissan_Cabstar_1_rc : RateTransition  Tag=mux_rc/StatePort  OutPortSampleTimeOpt=Inherit
  SpeedProfile : S-Function  Tag=SpeedProfile  LoadFcn=load('PrescanMotionData.mat')  FunctionName=sfun_SpeedProfile  Parameters=speedProfileUniqueID, timestep  EnableBusSupport=off  mask(SpeedProfile){speedProfileUniqueID=Demo_V2XStats_Intersection_1_cs_fcdd4688b7d5d124, timestep=1/20}
      mask prompts: speedProfileUniqueID "Speed Profile Unique ID"; timestep "MATLAB timestep:"
      mask help:
      | The speed profile block outputs the travelled distance, velocities and acceleration along a given path.
      |
      | For more information, please click Help.
      mask Help: eval('openHelp(312)')
      mask Display: image(imread('SpeedProfile.png'))
  Sum : Sum  Inputs=|++
  Sum3 : Sum  Inputs=|++
  Terminator_{1..6} (6 alike) : Terminator
  Unit Delay{1..2,4..7} (6 alike) : UnitDelay  SampleTime=-1
  V2X_2817_CAM_Create : MATLAB Function  LoadFcn=InitializeBus('CAM')  TreatAsAtomicUnit=on
  VehicleLength [m] : Constant  Value=5.836  OutDataTypeStr=int32
  VehicleWidth [m] : Constant  Value=2.376  OutDataTypeStr=int32
  "[deg to 0.01deg]" : Gain  Gain=100  OutDataTypeStr=int32
  "[deg to 0.1deg]" : Gain  Gain=10  OutDataTypeStr=int32
  "[deg to microdeg]" : Gain  Gain=10^6  OutDataTypeStr=int32
  "[deg to microdeg]1" : Gain  Gain=10^6  OutDataTypeStr=int32
  "[m to 0.1m]" : Gain  Gain=10  OutDataTypeStr=int32
  "[m to 0.1m]1" : Gain  Gain=10  OutDataTypeStr=int32
  "[m to cm]" : Gain  Gain=100  OutDataTypeStr=int32
  "[m to cm]1" : Gain  Gain=100  OutDataTypeStr=int32
  "[s to ms]" : Gain  Gain=1000  OutDataTypeStr=double
  int8_3 : Constant  Value=65536  OutDataTypeStr=double
  left_turning : Constant  Value=[0]  OutDataTypeStr=int8
  right_turning : Constant  Value=[0]  OutDataTypeStr=int8
  straight : Constant  Value=[0]  OutDataTypeStr=int8
  STATE_Nissan_Cabstar_1_bus : Outport  Tag=outport/StatePort  OutDataTypeStr=Bus: PRESCAN_STATEACTUATORDATA  PortDimensions=1  SampleTime=1/20
  V2X_Tx2817_CAM_Transmitter : Outport  Tag=outport/plugin/sfun_V2X_CAM_Transmitter  Port=2
  wires:
  Bit Set/1 -> Multiport Switch/2
  Multiport Switch/1 -> Data Type Conversion1/1
  Sum3/1 -> Multiport Switch/1
  [Target_Intention] -> Sum3/1
  Constant2/1 -> Sum3/2
  straight/1 -> Multiport Switch/3
  Bit Set1/1 -> Multiport Switch/4
  right_turning/1 -> Bit Set1/1
  left_turning/1 -> Bit Set/1
  Data Type Conversion1/1 -> V2X_2817_CAM_Create/10(exteriorLights)
  Constant1/1 -> Sum/2
  Sum/1 -> Multiport Switch1/1
  Path1/1 -> Multiport Switch1/3
  Path2/1 -> Multiport Switch1/4
  [Target_Intention] -> Sum/1
  Multiport Switch1/1 -> STATE_Nissan_Cabstar_1_rc/1
  Path/1 -> Multiport Switch1/2
  SpeedProfile/1 -> Path1/1, Path2/1, Path/1
  Math Function/1 -> Data Type Conversion/1
  "[s to ms]"/1 -> Math Function/1
  Date/Time Format Conversion/1(Generation_Time_Epoch) -> "[s to ms]"/1
  int8_3/1 -> Math Function/2
  Data Type Conversion/1 -> V2X_2817_CAM_Create/7(generationDeltaTime)
  Unit Delay6/1 -> V2X_2817_CAM_Create/3(velocity), Discrete Derivative/1
  "[m to cm]1"/1 -> Unit Delay6/1
  Discrete Derivative/1 -> V2X_2817_CAM_Create/4(longitudinalAcceleration)
  SELF_Demux/10(velocity [m/s]) -> "[m to cm]1"/1
  Unit Delay1/1 -> Mux/1
  "[deg to microdeg]"/1 -> Unit Delay1/1
  Unit Delay2/1 -> Mux/2
  "[deg to microdeg]1"/1 -> Unit Delay2/1
  Mux/1 -> V2X_2817_CAM_Create/1(gpsLatLon)
  SELF_Demux/7(GPS lat [deg]) -> "[deg to microdeg]"/1
  SELF_Demux/8(GPS long [deg]) -> "[deg to microdeg]1"/1
  "[deg to 0.1deg]"/1 -> Unit Delay4/1
  Unit Delay4/1 -> V2X_2817_CAM_Create/5(heading)
  SELF_Demux/11(heading [deg]) -> "[deg to 0.1deg]"/1
  "[m to cm]"/1 -> Unit Delay5/1
  Unit Delay5/1 -> V2X_2817_CAM_Create/2(altitude)
  SELF_Demux/9(GPS alt [m]) -> "[m to cm]"/1
  "[deg to 0.01deg]"/1 -> Unit Delay7/1
  Unit Delay7/1 -> V2X_2817_CAM_Create/6(yawRate)
  SELF_Demux/12(yaw rate [deg/s]) -> "[deg to 0.01deg]"/1
  VehicleLength [m]/1 -> "[m to 0.1m]"/1
  "[m to 0.1m]"/1 -> V2X_2817_CAM_Create/8(vehicleLength)
  VehicleWidth [m]/1 -> "[m to 0.1m]1"/1
  "[m to 0.1m]1"/1 -> V2X_2817_CAM_Create/9(vehicleWidth)
  STATE_Nissan_Cabstar_1_rc/1 -> STATE_Nissan_Cabstar_1_bus/1
  SELF_Nissan_Cabstar_1/1 -> SELF_Demux/1(SELF)
  V2X_2817_CAM_Create/1(message) -> V2X_Tx2817_CAM_Transmitter/1
  SELF_Demux/1(x [m]) -> Terminator_1/1
  SELF_Demux/2(y [m]) -> Terminator_2/1
  SELF_Demux/3(z [m]) -> Terminator_3/1
  SELF_Demux/4(rotx [deg]) -> Terminator_4/1
  SELF_Demux/5(roty [deg]) -> Terminator_5/1
  SELF_Demux/6(rotz [deg]) -> Terminator_6/1

== system Demo_V2XStats_Intersection_1_cs/PreScanTerminator ==
  Terminator : Terminator
  sfun_Terminator : S-Function  FunctionName=sfun_Terminator  Parameters=SampleTime  EnableBusSupport=off  mask(Legacy Function){SFunctionSpec=void prescan_terminator_outputFcn(void ** work1, PRESCAN_TERMINATORDATA y1[1]), SampleTime=TimeStep, ShowSpec=on}
      mask prompts: SampleTime "Sample time (-1 for inherited):"; ShowSpec "Display function specification"
      mask help:
      | This block allows you to call the legacy functions specified by the following Legacy Code Tool definition:
      | def.SFunctionName = 'sfun_Terminator';
      | def.OutputFcnSpec = 'void prescan_terminator_outputFcn(void ** work1, PRESCAN_TERMINATORDATA y1[1])';
      | def.StartFcnSpec = 'void prescan_terminator_startFcn(void ** work1)';
      | def.TerminateFcnSpec = 'void prescan_terminator_terminateFcn(void ** work1)';
      | def.HeaderFiles = {'prescan_terminator_data.h'};
      | def.HostLibFiles = {'sensorinterfaced.lib'};
      | def.IncPaths = {'src', 'C:\prescandev\vislibrary\vis\..\pimp\include\sensors\InterfaceRTW'};
      | def.SrcPaths = {'src'};
      | def.LibPaths = {'C:\\prescandev\\vislibrary_build\lib'};
      | def.SampleTime = 'parameterized';
      | def.Options.language = 'C';
      mask Help: <p>This block was generated automatically by the Legacy Code Tool. For detailed help on this tool, call<a href="matlab:legacy_code('help')"> legacy_code('help')</a>.</p>
      mask Callback ShowSpec:
      | if strcmp(get_param(gcbh, 'ShowSpec'), 'on')
      |   set_param(gcbh, 'MaskDisplay', sprintf('fprintf(''%s'');', get_param(gcbh, 'SFunctionSpec')));
      | else
      |   set_param(gcbh, 'MaskDisplay', sprintf('fprintf(''%s'');', get_param(gcbh, 'FunctionName')));
      | end
      mask Display: fprintf('void prescan_terminator_outputFcn(void ** work1, PRESCAN_TERMINATORDATA y1[1])');
  wires:
  sfun_Terminator/1 -> Terminator/1

== system Demo_V2XStats_Intersection_1_cs/SELF_Male_Regular_wSuitcase_1 ==
  Sensor : S-Function  FunctionName=sfun_SelfSensor  Parameters=UniqueID, TimeStep  EnableBusSupport=off  mask(PreScan Source Block: SELF){UniqueID=2658, TimeStep=1/20}
      mask prompts: UniqueID "Auto-Assigned: Unique ID"; TimeStep "Auto-Assigned: Upload Period [s]"
      mask help:
      | The SELF port shows (state) information of the actor itself. The outputs are position in the experiment's axis system and the GPS coordinates, and the object's absolute velocity and compass heading.
      |
      | For more information, please click Help.
      mask Help: eval('openHelp(462)')
      mask Display: image(imread('GPS.png'))
  SELF_Male_Regular_wSuitcase_1 : Outport  Tag=outport/SelfPort  OutDataTypeStr=Bus: PRESCAN_SELFSENSORDATA  PortDimensions=1  SampleTime=1/20
  wires:
  Sensor/1 -> SELF_Male_Regular_wSuitcase_1/1

== system Demo_V2XStats_Intersection_1_cs/SELF_Mazda_RX8_1 ==
  Sensor : S-Function  FunctionName=sfun_SelfSensor  Parameters=UniqueID, TimeStep  EnableBusSupport=off  mask(PreScan Source Block: SELF){UniqueID=7, TimeStep=1/20}
      mask prompts: UniqueID "Auto-Assigned: Unique ID"; TimeStep "Auto-Assigned: Upload Period [s]"
      mask help:
      | The SELF port shows (state) information of the actor itself. The outputs are position in the experiment's axis system and the GPS coordinates, and the object's absolute velocity and compass heading.
      |
      | For more information, please click Help.
      mask Help: eval('openHelp(462)')
      mask Display: image(imread('GPS.png'))
  SELF_Mazda_RX8_1 : Outport  Tag=outport/SelfPort  OutDataTypeStr=Bus: PRESCAN_SELFSENSORDATA  PortDimensions=1  SampleTime=1/20
  wires:
  Sensor/1 -> SELF_Mazda_RX8_1/1

== system Demo_V2XStats_Intersection_1_cs/SELF_Nissan_Cabstar_1 ==
  Sensor : S-Function  FunctionName=sfun_SelfSensor  Parameters=UniqueID, TimeStep  EnableBusSupport=off  mask(PreScan Source Block: SELF){UniqueID=10, TimeStep=1/20}
      mask prompts: UniqueID "Auto-Assigned: Unique ID"; TimeStep "Auto-Assigned: Upload Period [s]"
      mask help:
      | The SELF port shows (state) information of the actor itself. The outputs are position in the experiment's axis system and the GPS coordinates, and the object's absolute velocity and compass heading.
      |
      | For more information, please click Help.
      mask Help: eval('openHelp(462)')
      mask Display: image(imread('GPS.png'))
  SELF_Nissan_Cabstar_1 : Outport  Tag=outport/SelfPort  OutDataTypeStr=Bus: PRESCAN_SELFSENSORDATA  PortDimensions=1  SampleTime=1/20
  wires:
  Sensor/1 -> SELF_Nissan_Cabstar_1/1

== system Demo_V2XStats_Intersection_1_cs/STATE_Male_Regular_wSuitcase_1_bus ==
  STATE_Male_Regular_wSuitcase_1_bus : Inport  Tag=inport/StatePort  OutDataTypeStr=Bus: PRESCAN_STATEACTUATORDATA  PortDimensions=1  SampleTime=1/20  BusOutputAsStruct=on
  Actuator : S-Function  FunctionName=sfun_StateActuator  Parameters=UniqueID, TimeStep  EnableBusSupport=off  mask(PreScan Sink Block: State){UniqueID=2658, TimeStep=1/20}
      mask prompts: UniqueID "Auto-Assigned: Unique ID"; TimeStep "Auto-Assigned: Upload Period [s]"
      mask help:
      | The Actor State contains a vector signal of size (9x1), containing the following signals:
      |
      | -  Position    	(x,y,z)             	[m]
      | -  Velocity    	(vx,vy,vz)         	[m/s]
      | -  Angles       	(Roll, Pitch, Yaw)	[rad]
      |
      | The Actor state is defined in the global axis system.
      | The state is superponed on the Initial position defined in the GUI.
      |
      | For more information, please click Help.
      mask Help: eval('openHelp(222)')
      mask Display: image(imread('State.png'))
  wires:
  STATE_Male_Regular_wSuitcase_1_bus/1 -> Actuator/1

== system Demo_V2XStats_Intersection_1_cs/STATE_Mazda_RX8_1_bus ==
  STATE_Mazda_RX8_1_bus : Inport  Tag=inport/StatePort  OutDataTypeStr=Bus: PRESCAN_STATEACTUATORDATA  PortDimensions=1  SampleTime=1/20  BusOutputAsStruct=on
  Actuator : S-Function  FunctionName=sfun_StateActuator  Parameters=UniqueID, TimeStep  EnableBusSupport=off  mask(PreScan Sink Block: State){UniqueID=7, TimeStep=1/20}
      mask prompts: UniqueID "Auto-Assigned: Unique ID"; TimeStep "Auto-Assigned: Upload Period [s]"
      mask help:
      | The Actor State contains a vector signal of size (9x1), containing the following signals:
      |
      | -  Position    	(x,y,z)             	[m]
      | -  Velocity    	(vx,vy,vz)         	[m/s]
      | -  Angles       	(Roll, Pitch, Yaw)	[rad]
      |
      | The Actor state is defined in the global axis system.
      | The state is superponed on the Initial position defined in the GUI.
      |
      | For more information, please click Help.
      mask Help: eval('openHelp(222)')
      mask Display: image(imread('State.png'))
  wires:
  STATE_Mazda_RX8_1_bus/1 -> Actuator/1

== system Demo_V2XStats_Intersection_1_cs/STATE_Nissan_Cabstar_1_bus ==
  STATE_Nissan_Cabstar_1_bus : Inport  Tag=inport/StatePort  OutDataTypeStr=Bus: PRESCAN_STATEACTUATORDATA  PortDimensions=1  SampleTime=1/20  BusOutputAsStruct=on
  Actuator : S-Function  FunctionName=sfun_StateActuator  Parameters=UniqueID, TimeStep  EnableBusSupport=off  mask(PreScan Sink Block: State){UniqueID=10, TimeStep=1/20}
      mask prompts: UniqueID "Auto-Assigned: Unique ID"; TimeStep "Auto-Assigned: Upload Period [s]"
      mask help:
      | The Actor State contains a vector signal of size (9x1), containing the following signals:
      |
      | -  Position    	(x,y,z)             	[m]
      | -  Velocity    	(vx,vy,vz)         	[m/s]
      | -  Angles       	(Roll, Pitch, Yaw)	[rad]
      |
      | The Actor state is defined in the global axis system.
      | The state is superponed on the Initial position defined in the GUI.
      |
      | For more information, please click Help.
      mask Help: eval('openHelp(222)')
      mask Display: image(imread('State.png'))
  wires:
  STATE_Nissan_Cabstar_1_bus/1 -> Actuator/1

== system Demo_V2XStats_Intersection_1_cs/ScenarioEngine ==
  Clock : Clock
  sfun_ScenarioEngine : S-Function  FunctionName=sfun_ScenarioEngine  Parameters=TimeStep  EnableBusSupport=off
  wires:
  Clock/1 -> sfun_ScenarioEngine/1
